simulink model "hybird_p_car_21"  (R2021a)
settings: Solver=VariableStepAuto  StartTime=0.0  StopTime=2474  RelTol=1e-3
InitFcn:
  | m=1450;
  | g=9.81;
  | C=0.28;
  | frr=0.014;
  | et=0.97;
  | rw=0.29;
  | ig=1;
  | igf=2.5;
  | Vdc=400;
  | etmd=0.91;
  | RPMmax=12000;
  | Cmax=80;
  | k1=1;
  | k2=2;
libraries: autolibshared x1, pid_lib x1
settings Model: Creator=ab6273  LastModifiedBy=ae5046

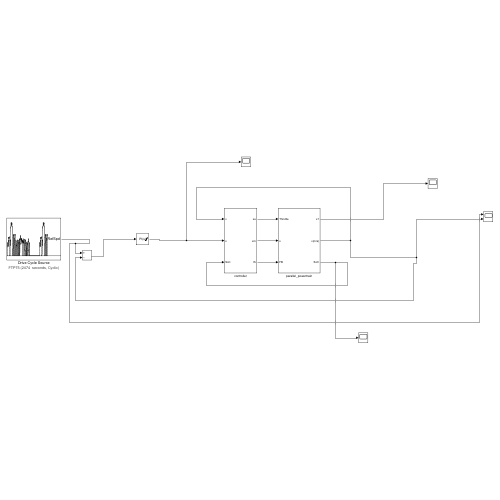
[thumbnail: Simulink's stored preview of the top-level diagram]
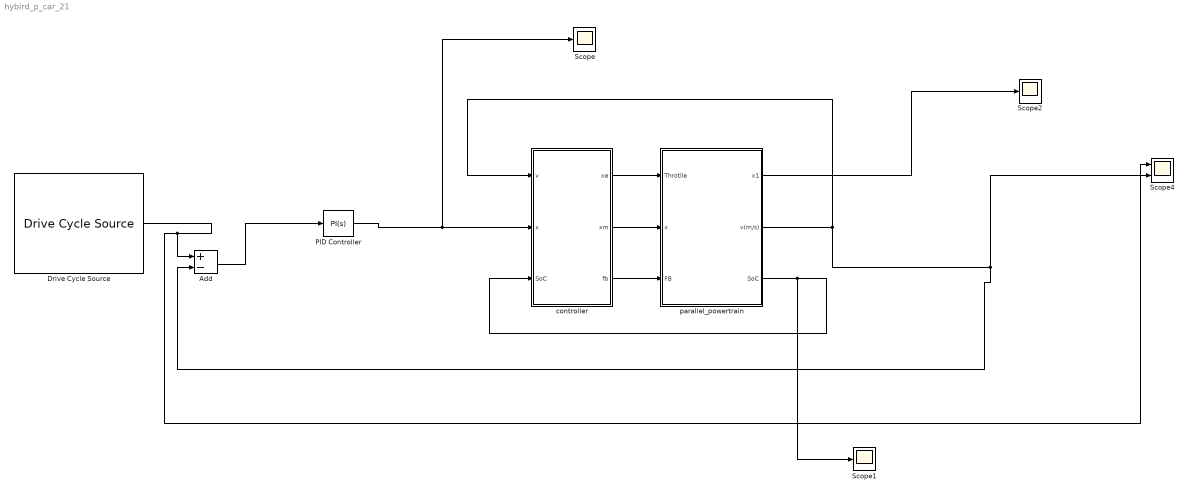
== system hybird_p_car_21 ==
  Add : Sum  Inputs=+-
  Drive Cycle Source : autolibshared/Drive Cycle Source  cycleVar=FTP75  fileVar=C:\Users\ab6273\OneDrive - Coventry University\Documents\6066MAA\Week 3- Control Engineering\HW3\WLTC_Class 3_Driving Cycle.xlsx  tfinal="2474  seconds, Cyclic"  cycleRepeat=on  outAccPort=off  outGearPort=off  gearList=No gear data  t_wot1=5  xdot_woto=0  xdot_wot1=30  t_wot2=20  xdot_wot2=0  t_wotend=30  srcUnit=m/s  outUnit=m/s  srcAccUnit=m/s/s  outAccUnit=m/s^2  dt=0  aMode=1  faultOption=off  velBnd=2  velBndUnit=mph  inUnit=m/s  timeBnd=1  failOption=off  stopSim=off  maxFaultCnt=10  maxFaultTime=2  maxTotFaultTime=15  traceOption=off  dtTrace=1  traceWindow=10  lastDCname=FTP75  lastOutUnit=mph  lastDT=0  lastTB=1  lastSB=2  forceCalcBound=off
  PID Controller : pid_lib/PID Controller  Controller=PI  Form=Parallel  TimeDomain=Continuous-time  UseExternalTs=off  SampleTime=-1  IntegratorMethod=Forward Euler  FilterMethod=Forward Euler  ControllerParametersSource=internal  P=0.4  I=0.1  D=0  N=100  UseFilter=on  TunerSelectOption=Transfer Function Based (PID Tuner App)  InitialConditionSource=internal  InitialConditionForIntegrator=0  InitialConditionForFilter=0  DifferentiatorICPrevScaledInput=0  ExternalReset=none  TrackingMode=off  Kt=1  LimitOutput=on  SatLimitsSource=internal  UpperSaturationLimit=1  LowerSaturationLimit=-1  LinearizeAsGain=on  AntiWindupMode=back-calculation  Kb=0.12  POutMin=[]  POutMax=[]  IOutMin=[]  IOutMax=[]  DOutMin=[]  DOutMax=[]  NOutMin=[]  NOutMax=[]  SumOutMin=[]  SumOutMax=[]  SaturationOutMin=[]  SaturationOutMax=[]  PParamMin=[]  PParamMax=[]  IParamMin=[]  IParamMax=[]  DParamMin=[]  DParamMax=[]  NParamMin=[]  NParamMax=[]  KbParamMin=[]  KbParamMax=[]  KtParamMin=[]  KtParamMax=[]  KbOutMin=[]  KbOutMax=[]  KtOutMin=[]  KtOutMax=[]  IntegratorOutMin=[]  IntegratorOutMax=[]  FilterOutMin=[]  FilterOutMax=[]  SumI1OutMin=[]  SumI1OutMax=[]  SumI2OutMin=[]  SumI2OutMax=[]  SumI3OutMin=[]  SumI3OutMax=[]  SumI4OutMin=[]  SumI4OutMax=[]  SumDOutMin=[]  SumDOutMax=[]  DifferentiatorOutMin=[]  DifferentiatorOutMax=[]  FilterDiffOutCoefMin=[]  FilterDiffOutCoefMax=[]  ReciprocalOutMin=[]  ReciprocalOutMax=[]  SumDenOutMin=[]  SumDenOutMax=[]  SumNumOutMin=[]  SumNumOutMax=[]  DivideOutMin=[]  DivideOutMax=[]  UdiffTsProdOutMin=[]  UdiffTsProdOutMax=[]  NTsProdOutMin=[]  NTsProdOutMax=[]  UintegralTsProdOutMin=[]  UintegralTsProdOutMax=[]  UngainTsProdOutMin=[]  UngainTsProdOutMax=[]  IntegratorContinuousStateAttributes=''  IntegratorStateMustResolveToSignalObject=off  IntegratorRTWStateStorageClass=Auto  FilterContinuousStateAttributes=''  FilterStateMustResolveToSignalObject=off  FilterRTWStateStorageClass=Auto  ParallelPVariant=InternalParameters  IdealPVariant=Disabled  IVariant=InternalParameters  DVariant=Disabled  IntegratorVariant=Continuous  SatVariant=Enabled  AWVariant=BackCalculation  PCopyVariant=Disabled  TRVariant=Disabled  FdbkBlocksVariant=Forward  IdealPFdbkVariant=Disabled  SatFdbkVariant=Disabled  DerivativeFilterVariant=Disabled  NVariant=Disabled  NCopyVariant=Disabled_SignalSpec  FilterICVariant=Disabled  IntegratorICVariant=InternalICs  ExternalResetVariant=Disabled  TRSumVariant=Passthrough  SumFdbkVariant=Disabled  SumVariant=Sum_PI  TsampFilterVariant=InternalTs  TsampNgainVariant=Passthrough  TsampIntegralVariant=Disabled_SignalSpec  ExternalSaturationOutDataTypeStr=Inherit: Same as second input
  Scope : Scope
  Scope1 : Scope
  Scope2 : Scope
  Scope4 : Scope  NumInputPorts=2
  controller : Subsystem
  parallel_powertrain : Subsystem
  wires:
  Add/1 -> PID Controller/1
  Drive Cycle Source/1 -> Add/1, Scope4/1
  parallel_powertrain/2(v(m/s)) -> Scope4/2, Add/2, controller/1(v)
  parallel_powertrain/1(x1) -> Scope2/1
  controller/1(xe) -> parallel_powertrain/1(Throtlle)
  controller/2(xm) -> parallel_powertrain/2(x)
  controller/3(fb) -> parallel_powertrain/3(FB)
  PID Controller/1 -> Scope/1, controller/2(x)
  parallel_powertrain/3(SoC) -> Scope1/1, controller/3(SoC)

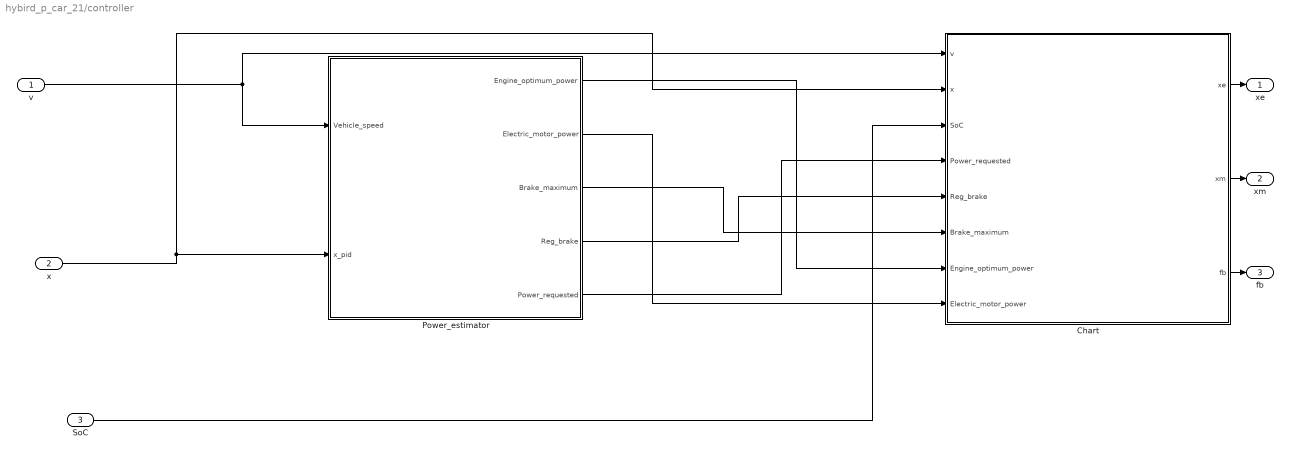
== system hybird_p_car_21/controller ==
  v : Inport
  x : Inport  Port=2
  SoC : Inport  Port=3
  Chart : Stateflow chart  TreatAsAtomicUnit=on
  Power_estimator : Subsystem
  xe : Outport
  xm : Outport  Port=2
  fb : Outport  Port=3
  wires:
  Power_estimator/5(Power_requested) -> Chart/4(Power_requested)
  v/1 -> Chart/1(v), Power_estimator/1(Vehicle_speed)
  x/1 -> Chart/2(x), Power_estimator/2(x_pid)
  Chart/2(xm) -> xm/1
  Power_estimator/1(Engine_optimum_power) -> Chart/7(Engine_optimum_power)
  Power_estimator/3(Brake_maximum) -> Chart/6(Brake_maximum)
  Power_estimator/4(Reg_brake) -> Chart/5(Reg_brake)
  Power_estimator/2(Electric_motor_power) -> Chart/8(Electric_motor_power)
  Chart/1(xe) -> xe/1
  Chart/3(fb) -> fb/1
  SoC/1 -> Chart/3(SoC)

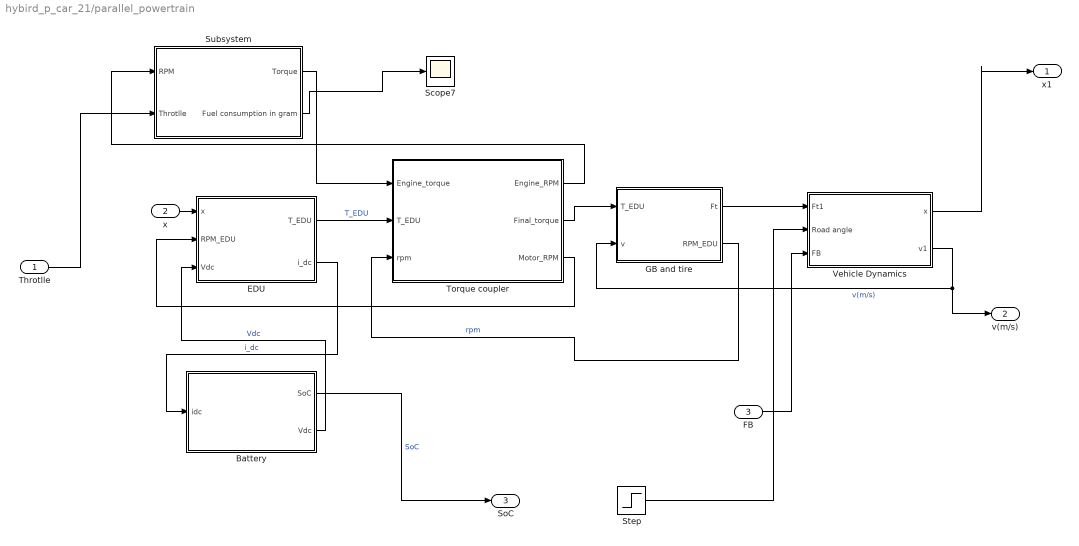
== system hybird_p_car_21/parallel_powertrain ==
  Throtlle : Inport
  x : Inport  Port=2
  FB : Inport  Port=3
  Battery : Subsystem
  EDU : Subsystem
  GB and tire : Subsystem
  Scope7 : Scope
  Step : Step  Time=1000  After=0  SampleTime=0
  Subsystem : Subsystem
  Torque coupler : Subsystem
  Vehicle Dynamics : Subsystem
  x1 : Outport
  v(m/s) : Outport  Port=2
  SoC : Outport  Port=3
  wires:
  Vehicle Dynamics/1(x) -> x1/1
  Vehicle Dynamics/2(v1) -> v(m/s)/1, GB and tire/2(v)  "v(m/s)"
  Throtlle/1 -> Subsystem/2(Throtlle)
  Subsystem/2(Fuel consumption in gram) -> Scope7/1
  EDU/2(i_dc) -> Battery/1(idc)  "i_dc"
  Step/1 -> Vehicle Dynamics/2(Road angle)
  x/1 -> EDU/1(x)
  Torque coupler/3(Motor_RPM) -> EDU/2(RPM_EDU)
  Battery/2(Vdc) -> EDU/3(Vdc)  "Vdc"
  Battery/1(SoC) -> SoC/1  "SoC"
  GB and tire/1(Ft) -> Vehicle Dynamics/1(Ft1)
  Torque coupler/2(Final_torque) -> GB and tire/1(T_EDU)
  FB/1 -> Vehicle Dynamics/3(FB)
  EDU/1(T_EDU) -> Torque coupler/2(T_EDU)  "T_EDU"
  GB and tire/2(RPM_EDU) -> Torque coupler/3(rpm)  "rpm"
  Torque coupler/1(Engine_RPM) -> Subsystem/1(RPM)
  Subsystem/1(Torque) -> Torque coupler/1(Engine_torque)

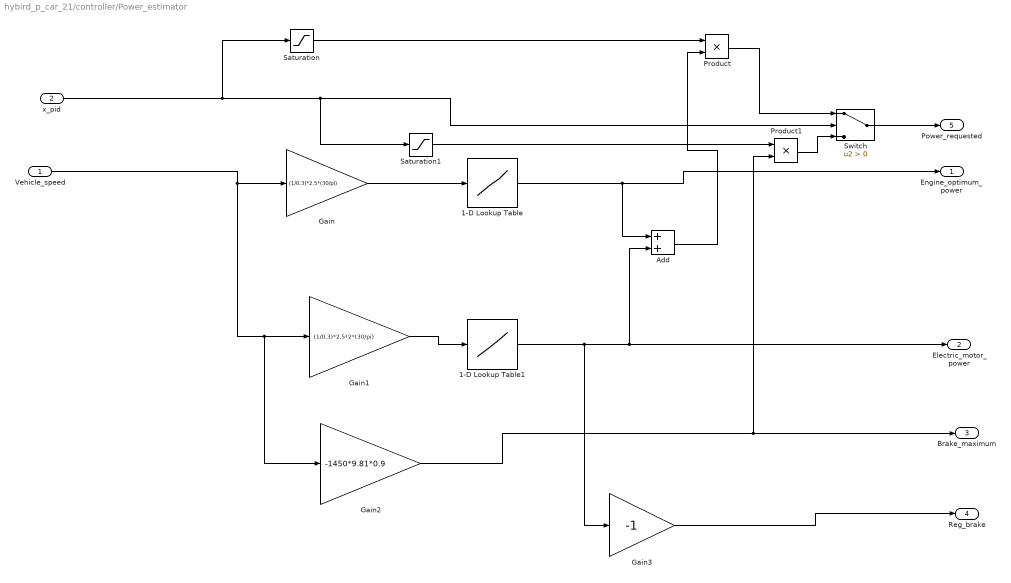
== system hybird_p_car_21/controller/Power_estimator ==
  Vehicle_speed : Inport
  x_pid : Inport  Port=2
  1-D Lookup Table : Lookup_n-D  NumberOfTableDimensions=1  BreakpointsForDimension1=[0;950;1000;1200;1500;1600;2000;2600;3600;4300;5000;6000;6500;8000]  Table=[0;0;1000;5000;10000;20000;40000;70000;100000;130000;130000;113097;0;0]  InternalRulePriority=Speed  RndMeth=Simplest  InputSameDT=on
  1-D Lookup Table1 : Lookup_n-D  NumberOfTableDimensions=1  BreakpointsForDimension1=[0;1200;2400;3600;4800;6000;7200;8400;9600;10800;12000;13200;14400]  Table=[0;32656;65312;97968;130624;130624;130372.8;131000.8;130624;131126.39999999999;130624;131252;131126.39999999999]  InternalRulePriority=Speed  RndMeth=Simplest  InputSameDT=on
  Add : Sum
  Gain : Gain  Gain=(1/0.3)*2.5*(30/pi)
  Gain1 : Gain  Gain=(1/0.3)*2.5*2*(30/pi)
  Gain2 : Gain  Gain=-1450*9.81*0.9
  Gain3 : Gain  Gain=-1
  Product : Product
  Product1 : Product
  Saturation : Saturate  UpperLimit=1  LowerLimit=0
  Saturation1 : Saturate  UpperLimit=0  LowerLimit=-1
  Switch : Switch  Criteria=u2 > Threshold
  Engine_optimum_power : Outport
  Electric_motor_power : Outport  Port=2
  Brake_maximum : Outport  Port=3
  Reg_brake : Outport  Port=4
  Power_requested : Outport  Port=5
  wires:
  Gain3/1 -> Reg_brake/1
  Gain2/1 -> Brake_maximum/1, Product1/2
  1-D Lookup Table1/1 -> Gain3/1, Electric_motor_power/1, Add/2
  Vehicle_speed/1 -> Gain2/1, Gain1/1, Gain/1
  1-D Lookup Table/1 -> Engine_optimum_power/1, Add/1
  Gain1/1 -> 1-D Lookup Table1/1
  Gain/1 -> 1-D Lookup Table/1
  Add/1 -> Product/2
  x_pid/1 -> Saturation/1, Saturation1/1, Switch/2
  Switch/1 -> Power_requested/1
  Product1/1 -> Switch/3
  Product/1 -> Switch/1
  Saturation/1 -> Product/1
  Saturation1/1 -> Product1/1

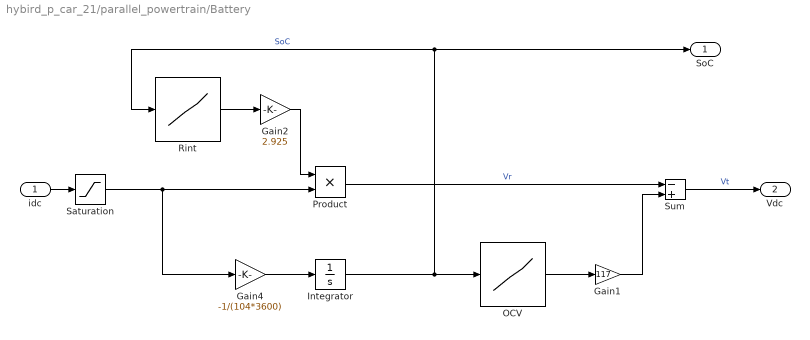
== system hybird_p_car_21/parallel_powertrain/Battery ==
  idc : Inport
  Gain1 : Gain  Gain=117
  Gain2 : Gain  Gain=2.925
  Gain4 : Gain  Gain=-1/(104*3600)
  Integrator : Integrator  InitialCondition=1
  OCV : Lookup_n-D  NumberOfTableDimensions=1  BreakpointsForDimension1=|  Table=|  InternalRulePriority=Speed  RndMeth=Simplest  InputSameDT=on
      BreakpointsForDimension1=|
      | [0
      | 0.006648936
      | 0.021276596
      | 0.053191489
      | 0.087765957
      | 0.186170213
      | 0.308510638
      | 0.457446809
      | 0.590425532
      | 0.710106383
      | 0.813829787
      | 0.909574468
      | 0.998670213
      | ]
      Table=|
      | [3.002620087
      | 3.201746725
      | 3.390393013
      | 3.561572052
      | 3.610480349
      | 3.659388646
      | 3.701310044
      | 3.736244541
      | 3.795633188
      | 3.865502183
      | 3.952838428
      | 4.050655022
      | 4.162445415
      | ]
  Product : Product
  Rint : Lookup_n-D  NumberOfTableDimensions=1  BreakpointsForDimension1=|  Table=|  InternalRulePriority=Speed  RndMeth=Simplest  InputSameDT=on
      BreakpointsForDimension1=|
      | [0
      | 0.041223404
      | 0.099734043
      | 0.200797872
      | 0.39893617
      | 0.599734043
      | 0.800531915
      | 1
      | ]
      Table=|
      | [0.135819057
      | 0.128988915
      | 0.091367148
      | 0.079722316
      | 0.069868996
      | 0.070764752
      | 0.074347777
      | 0.057328407
      | ]
  Saturation : Saturate  UpperLimit=inf  LowerLimit=0
  Sum : Sum  Inputs=-+
  SoC : Outport
  Vdc : Outport  Port=2
  wires:
  Sum/1 -> Vdc/1  "Vt"
  Gain1/1 -> Sum/2
  Product/1 -> Sum/1  "Vr"
  OCV/1 -> Gain1/1
  Rint/1 -> Gain2/1
  Gain2/1 -> Product/1
  idc/1 -> Saturation/1
  Integrator/1 -> SoC/1, Rint/1, OCV/1  "SoC"
  Gain4/1 -> Integrator/1
  Saturation/1 -> Gain4/1, Product/2

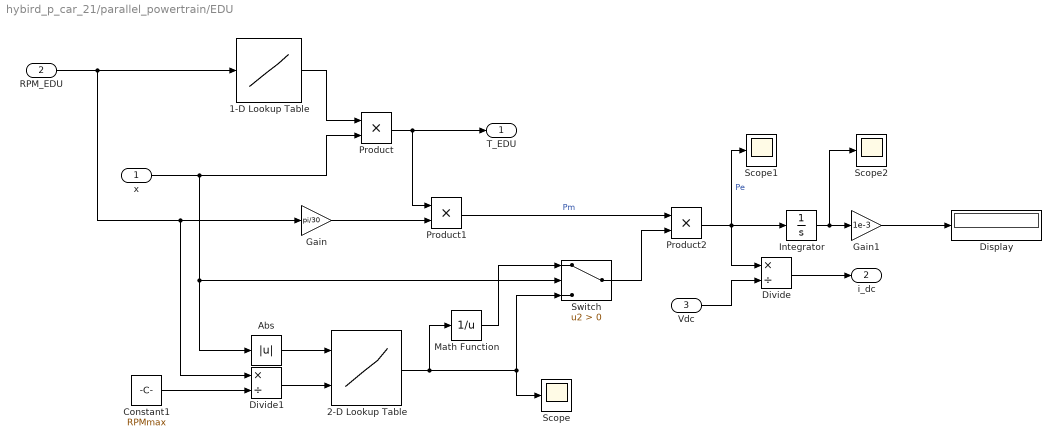
== system hybird_p_car_21/parallel_powertrain/EDU ==
  x : Inport
  RPM_EDU : Inport  Port=2
  Vdc : Inport  Port=3
  1-D Lookup Table : Lookup_n-D  NumberOfTableDimensions=1  BreakpointsForDimension1=|  Table=|  InternalRulePriority=Speed  RndMeth=Simplest  InputSameDT=on
      BreakpointsForDimension1=|
      | [0
      | 500
      | 1000
      | 1500
      | 2000
      | 2387
      | 3000
      | 4000
      | 5000
      | 6000
      | 7000
      | 8000
      | 9000
      | 10000
      | 11000
      | 11100
      | 12000
      | ]
      Table=|
      | [400
      | 400
      | 400
      | 400
      | 400
      | 400
      | 318.31
      | 238.73
      | 190.99
      | 159.15
      | 136.42
      | 119.37
      | 106.10
      | 95.49
      | 86.81
      | 0
      | 0
      | ]
  2-D Lookup Table : Lookup_n-D  BreakpointsForDimension1=[0:0.1:1]  BreakpointsForDimension2=[0:0.1:1]  Table=|  InternalRulePriority=Speed  RndMeth=Simplest  InputSameDT=on
      | [0.9	0.8245	0.821274236	0.808389063	0.597551308	0.467557578	0.359250515	0.311171352	0.276214917	0.241993553	0.139250965
      | 0.9215	0.97	0.966204983	0.951045956	0.703001538	0.550067739	0.422647665	0.366083944	0.324958726	0.284698297	0.163824664
      | 0.9215	0.97	0.97	0.965120507	0.944479504	0.92081464	0.84529533	0.732167887	0.649917453	0.569396595	0.327649328
      | 0.9215	0.97	0.97	0.97	0.953738777	0.932919866	0.881645654	0.867028235	0.868747783	0.854094892	0.491473993
      | 0.91852093	0.966864137	0.97	0.97	0.960084237	0.941224296	0.917995978	0.886276783	0.875321322	0.85852819	0.607991095
      | 0.9075065	0.95527	0.97	0.969374488	0.96222553	0.947628327	0.925528376	0.901055615	0.881894861	0.862961487	0.700854417
      | 0.886479941	0.93313678	0.960922964	0.95929013	0.963018495	0.950793534	0.933060774	0.906895014	0.886331305	0.867394784	0.793717738
      | 0.893731423	0.940769919	0.951592737	0.949205773	0.961549062	0.953381895	0.937964411	0.912734413	0.889699201	0.871095296	0.856768318
      | 0.869628401	0.915398317	0.94150838	0.94	0.956903166	0.954816567	0.942868048	0.917392061	0.893067098	0.874795808	0.860193414
      | 0.840964375	0.885225658	0.94	0.94	0.949339898	0.954983355	0.944502472	0.922049709	0.896411995	0.878496321	0.863618509
      | 0.776546979	0.817417872	0.94	0.94	0.943409404	0.954516201	0.946136896	0.926264205	0.899756892	0.881408077	0.867043605
      |  ]
      settings: InputPortMap=u0,u1
  Abs : Abs
  Constant1 : Constant  Value=RPMmax
  Display : Display
  Divide : Product  Inputs=*/
  Divide1 : Product  Inputs=*/
  Gain : Gain  Gain=pi/30
  Gain1 : Gain  Gain=1e-3
  Integrator : Integrator
  Math Function : Math  Operator=reciprocal  SaturateOnIntegerOverflow=on
  Product : Product
  Product1 : Product
  Product2 : Product
  Scope : Scope
  Scope1 : Scope
  Scope2 : Scope
  Switch : Switch  Criteria=u2 > Threshold
  T_EDU : Outport
  i_dc : Outport  Port=2
  wires:
  1-D Lookup Table/1 -> Product/1
  Product/1 -> Product1/1, T_EDU/1
  RPM_EDU/1 -> 1-D Lookup Table/1, Gain/1, Divide1/1
  Gain/1 -> Product1/2
  Product1/1 -> Product2/1  "Pm"
  Switch/1 -> Product2/2
  x/1 -> Abs/1, Switch/2, Product/2
  Product2/1 -> Divide/1, Integrator/1, Scope1/1  "Pe"
  Vdc/1 -> Divide/2
  Divide/1 -> i_dc/1
  Divide1/1 -> 2-D Lookup Table/2
  Constant1/1 -> Divide1/2
  Abs/1 -> 2-D Lookup Table/1
  2-D Lookup Table/1 -> Scope/1, Switch/3, Math Function/1
  Math Function/1 -> Switch/1
  Integrator/1 -> Scope2/1, Gain1/1
  Gain1/1 -> Display/1

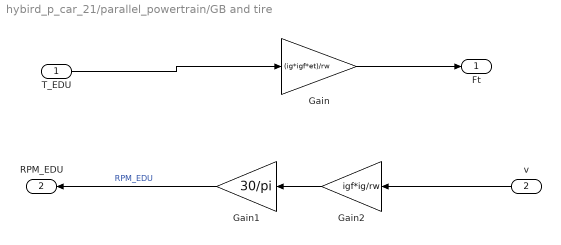
== system hybird_p_car_21/parallel_powertrain/GB and tire ==
  T_EDU : Inport
  v : Inport  Port=2
  Gain : Gain  Gain=(ig*igf*et)/rw
  Gain1 : Gain  Gain=30/pi
  Gain2 : Gain  Gain=igf*ig/rw
  Ft : Outport
  RPM_EDU : Outport  Port=2
  wires:
  Gain2/1 -> Gain1/1
  Gain/1 -> Ft/1
  Gain1/1 -> RPM_EDU/1  "RPM_EDU"
  v/1 -> Gain2/1
  T_EDU/1 -> Gain/1

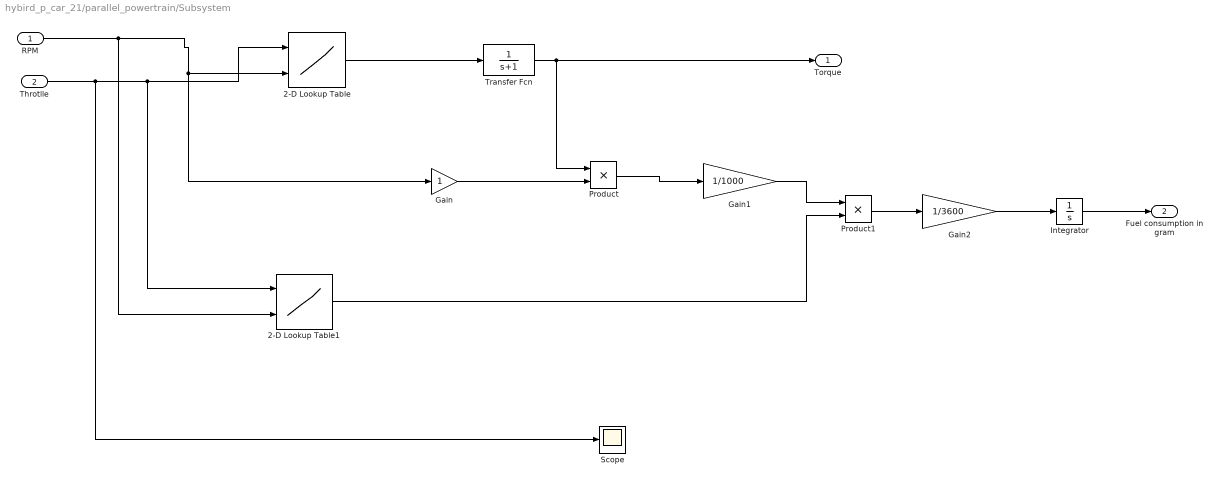
== system hybird_p_car_21/parallel_powertrain/Subsystem ==
  RPM : Inport
  Throtlle : Inport  Port=2
  2-D Lookup Table : Lookup_n-D  BreakpointsForDimension1=[0.1;0.2;0.4;0.6;0.8;1]  BreakpointsForDimension2=[1000;2000;2500;3000;3500;4000;4500;4750;5320;5800;6000]  Table=[0 0 0 0 0 0 0 0 0 0 0;65.400000000000006 45.700000000000003 37.200000000000003 27.800000000000001 23.5 19.100000000000001 15.6 11.9 0 0 0;98 85.900000000000006 77.599999999999994 69.299999999999997 63.799999999999997 56.899999999999999 50.5 46 32.200000000000003 21.300000000000001 17.399999999999999;106 103.59999999999999 96.700000000000003 89.599999999999994 86.400000000000006 80.900000000000006 74 69.799999999999997 55.700000000000003 45.799999999999997 41.200000000000003;115.3 121.90000000000001 127.3 131.09999999999999 120.5 125.5 124.5 125.09999999999999 118.8 109.59999999999999 104.7;117.2 123.59999999999999 129.09999999999999 132.09999999999999 134.30000000000001 137.19999999999999 134.80000000000001 135.19999999999999 129 119.3 113.09999999999999]  InternalRulePriority=Speed  RndMeth=Simplest  InputSameDT=on
      settings: InputPortMap=u0,u1
  2-D Lookup Table1 : Lookup_n-D  BreakpointsForDimension1=[0.1;0.2;0.4;0.6;0.8;1]  BreakpointsForDimension2=[1000;2000;2500;3000;3500;4000;4500;4750;5320;5800;6000]  Table=[426.4046 471.0416 430.0417 518.7181 643.4765 810.9169000000001 971.3416 1050 1100 1150 1200;243.3556 271.9792 297.6581 332.2183 382.7842 449.4108 517.1757 640.501 660 680 700;221.8311 222.448 231.4663 238.9684 252.4381 268.6577 290.0927 305.8607 379.2565 487.9831 540.9734;222.0534 216.825 221.3162 224.0502 230.7725 239.2966 258.3073 259.5352 290.0497 331.0725 356.0068;226.4276 215.5953 219.2097 221.0032 219.8004 234.1577 255.8003 257.1846 275.1281 311.0458 305.842;228.8846 227.9702 227.9965 224.2643 229.6245 255.9767 266.1145 278.1351 288.2523 303.7707 313.966]  InternalRulePriority=Speed  RndMeth=Simplest  InputSameDT=on
      settings: InputPortMap=u0,u1
  Gain : Gain
  Gain1 : Gain  Gain=1/1000
  Gain2 : Gain  Gain=1/3600
  Integrator : Integrator
  Product : Product
  Product1 : Product
  Scope : Scope
  Transfer Fcn : TransferFcn  Denominator=[1 1]
  Torque : Outport
  Fuel consumption in gram : Outport  Port=2
  wires:
  Throtlle/1 -> Scope/1, 2-D Lookup Table1/1, 2-D Lookup Table/1
  RPM/1 -> 2-D Lookup Table1/2, 2-D Lookup Table/2, Gain/1
  2-D Lookup Table/1 -> Transfer Fcn/1
  Transfer Fcn/1 -> Product/1, Torque/1
  Gain/1 -> Product/2
  Product/1 -> Gain1/1
  Gain1/1 -> Product1/1
  2-D Lookup Table1/1 -> Product1/2
  Product1/1 -> Gain2/1
  Gain2/1 -> Integrator/1
  Integrator/1 -> Fuel consumption in gram/1

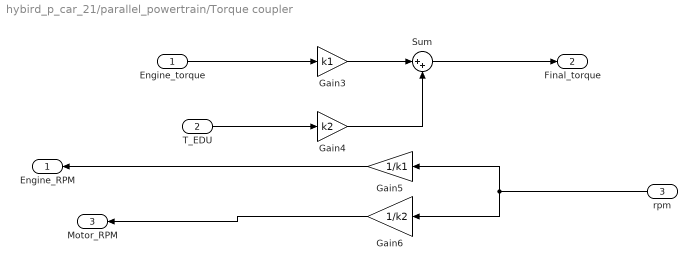
== system hybird_p_car_21/parallel_powertrain/Torque coupler ==
  Engine_torque : Inport
  T_EDU : Inport  Port=2
  rpm : Inport  Port=3
  Gain3 : Gain  Gain=k1
  Gain4 : Gain  Gain=k2
  Gain5 : Gain  Gain=1/k1
  Gain6 : Gain  Gain=1/k2
  Sum : Sum  Inputs=|++
  Engine_RPM : Outport
  Final_torque : Outport  Port=2
  Motor_RPM : Outport  Port=3
  wires:
  rpm/1 -> Gain6/1, Gain5/1
  Engine_torque/1 -> Gain3/1
  Sum/1 -> Final_torque/1
  Gain3/1 -> Sum/1
  Gain5/1 -> Engine_RPM/1
  Gain6/1 -> Motor_RPM/1
  T_EDU/1 -> Gain4/1
  Gain4/1 -> Sum/2

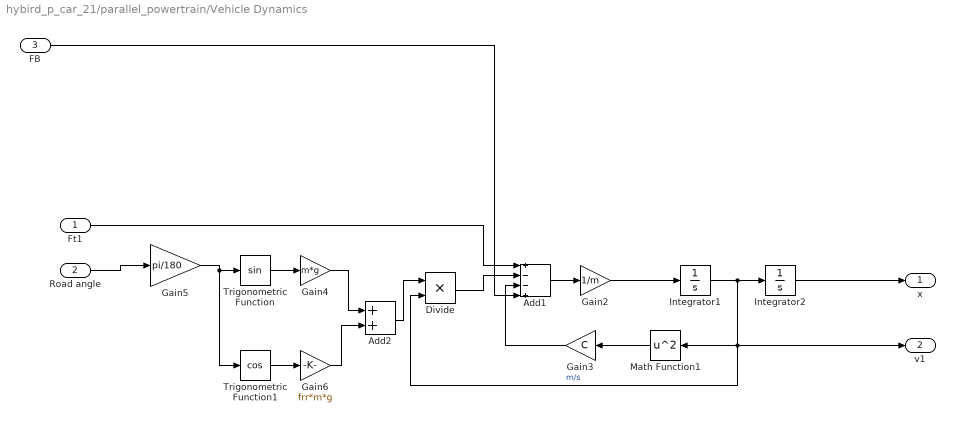
== system hybird_p_car_21/parallel_powertrain/Vehicle Dynamics ==
  Ft1 : Inport
  Road angle : Inport  Port=2
  FB : Inport  Port=3
  Add1 : Sum  Inputs=+--+
  Add2 : Sum
  Divide : Product
  Gain2 : Gain  Gain=1/m
  Gain3 : Gain  Gain=C
  Gain4 : Gain  Gain=m*g
  Gain5 : Gain  Gain=pi/180
  Gain6 : Gain  Gain=frr*m*g
  Integrator1 : Integrator
  Integrator2 : Integrator
  Math Function1 : Math  Operator=square  SaturateOnIntegerOverflow=on
  Trigonometric Function : Trigonometry
  Trigonometric Function1 : Trigonometry  Operator=cos
  x : Outport
  v1 : Outport  Port=2
  wires:
  Trigonometric Function/1 -> Gain4/1
  Integrator2/1 -> x/1
  Add2/1 -> Divide/1
  Add1/1 -> Gain2/1
  Gain5/1 -> Trigonometric Function1/1, Trigonometric Function/1
  Gain2/1 -> Integrator1/1
  Ft1/1 -> Add1/1
  Road angle/1 -> Gain5/1
  Integrator1/1 -> Divide/2, v1/1, Math Function1/1, Integrator2/1  "m/s"
  Gain6/1 -> Add2/2
  Gain4/1 -> Add2/1
  Math Function1/1 -> Gain3/1
  Gain3/1 -> Add1/3
  Trigonometric Function1/1 -> Gain6/1
  Divide/1 -> Add1/2
  FB/1 -> Add1/4

== stateflow chart hybird_p_car_21/controller/Chart ==
  state Traction
    state LOWSPEED
      xe=0;
      xm=x;
      fb=0;
    state HIGHSPEED
      xe=x;
      xm=x;
      fb=0;
    (default) -> LOWSPEED
    HIGHSPEED -> LOWSPEED : [v>=3]
    LOWSPEED -> HIGHSPEED : [v<=3]
  state Idle
    xe=0;
    xm=0;
    fb=0;
  state Braking
    state REGBRAKING
      xe=0;
      xm=x;
      fb=0;
    (default) -> REGBRAKING
  (default) -> Idle
  Idle -> Traction [order 1] : [x>0.01]
  Braking -> Idle : [x>-0.01]
  Traction -> Idle : [x<0.01]
  Idle -> Braking [order 2] : [x<-0.01]
  data: xe output; xm output; fb output; v input; x input; SoC input; Power_requested input; Reg_brake input; Brake_maximum input; Engine_optimum_power input; Electric_motor_power input
